simulink model "CTRL_SPECCTRL_FF_RSTOP_test"  (R2024b)
settings: Solver=VariableStepAuto  StartTime=0.0  StopTime=10.0  RelTol=1e-3
libraries: CTRL_SPECCTRL_FF_RSTOP x1
settings Model: Creator=blatak  LastModifiedBy=blatak

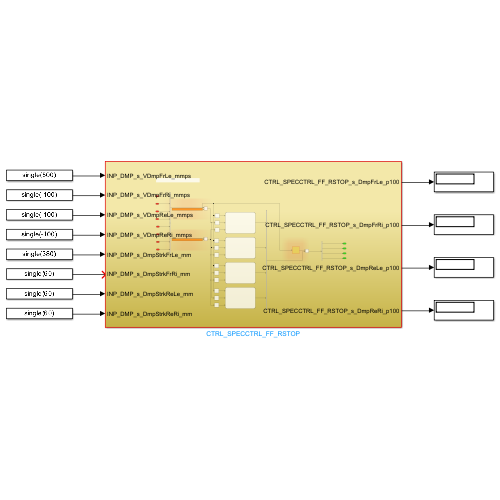
[thumbnail: Simulink's stored preview of the top-level diagram]
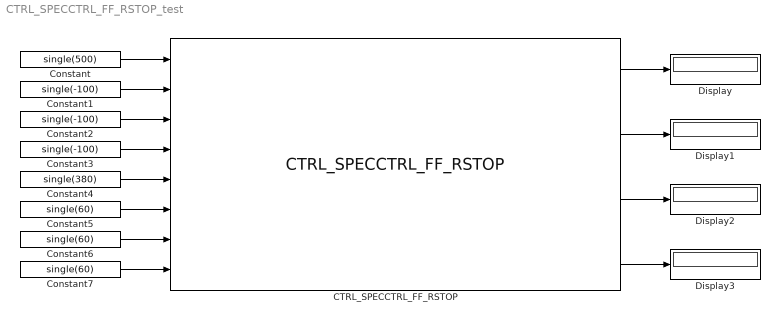
== system CTRL_SPECCTRL_FF_RSTOP_test ==
  CTRL_SPECCTRL_FF_RSTOP : CTRL_SPECCTRL_FF_RSTOP/CTRL_SPECCTRL_FF_RSTOP  SystemSampleTime=-1  VariantActivationTime=update diagram  AllowFlexibleInterface=on  Latency=0  AutoFrameSizeCalculation=off
  Constant : Constant  Value=single(500)
  Constant1 : Constant  Value=single(-100)
  Constant2 : Constant  Value=single(-100)
  Constant3 : Constant  Value=single(-100)
  Constant4 : Constant  Value=single(380)
  Constant5 : Constant  Value=single(60)
  Constant6 : Constant  Value=single(60)
  Constant7 : Constant  Value=single(60)
  Display{,1..3} (4 alike) : Display
  wires:
  CTRL_SPECCTRL_FF_RSTOP/1 -> Display/1
  CTRL_SPECCTRL_FF_RSTOP/2 -> Display1/1
  CTRL_SPECCTRL_FF_RSTOP/3 -> Display2/1
  CTRL_SPECCTRL_FF_RSTOP/4 -> Display3/1
  Constant/1 -> CTRL_SPECCTRL_FF_RSTOP/1
  Constant1/1 -> CTRL_SPECCTRL_FF_RSTOP/2
  Constant2/1 -> CTRL_SPECCTRL_FF_RSTOP/3
  Constant3/1 -> CTRL_SPECCTRL_FF_RSTOP/4
  Constant4/1 -> CTRL_SPECCTRL_FF_RSTOP/5
  Constant5/1 -> CTRL_SPECCTRL_FF_RSTOP/6
  Constant6/1 -> CTRL_SPECCTRL_FF_RSTOP/7
  Constant7/1 -> CTRL_SPECCTRL_FF_RSTOP/8
